simulink model "glucose"  (R2022a)
settings: Solver=VariableStepAuto  StartTime=0.0  StopTime=182  RelTol=1e-3
model workspace: external: MATLAB File parameters.m (data not in the file)
undefined symbols (not defined in the file): G0, Gb, Ib, insuline, k, Sg, Si, time
settings Model: Creator=bigba  LastModifiedBy=bigba

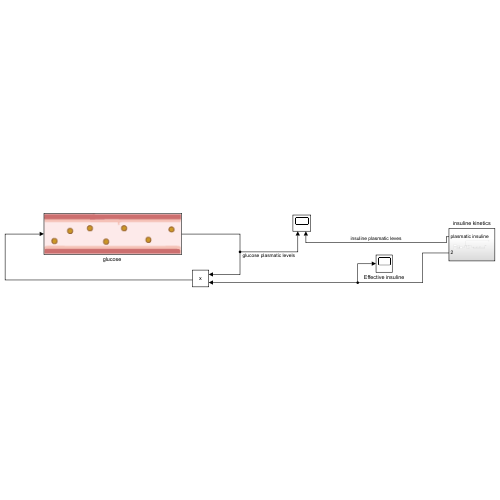
[thumbnail: Simulink's stored preview of the top-level diagram]
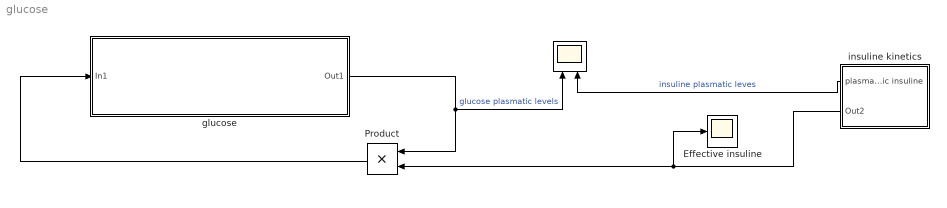
== system glucose ==
  " " : Scope  NumInputPorts=2
  Effective insuline : Scope
  Product : Product
  "glucose " : Subsystem
      mask Display: image('$imagefile'); % Use "Edit Image" on toolstrip to change.
  insuline kinetics : Subsystem
  wires:
  "glucose "/1(Out1) -> Product/1, " "/1  "glucose plasmatic levels"
  Product/1 -> "glucose "/1(In1)
  insuline kinetics/2(Out2) -> Product/2, Effective insuline/1
  insuline kinetics/1(plasmatic insuline) -> " "/2  "insuline plasmatic leves"

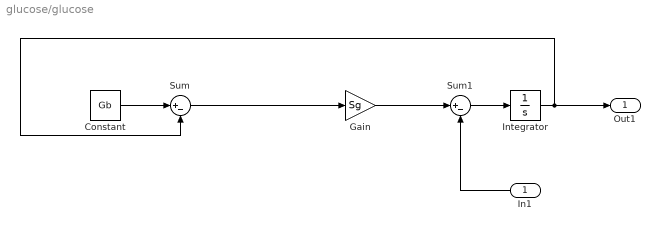
== system glucose/glucose  ==
  In1 : Inport
  Constant : Constant  Value=Gb
  Gain : Gain  Gain=Sg
  Integrator : Integrator  InitialCondition=G0
  Sum : Sum  Inputs=|+-
  Sum1 : Sum  Inputs=|+-
  Out1 : Outport
  wires:
  Gain/1 -> Sum1/1
  In1/1 -> Sum1/2
  Integrator/1 -> Out1/1, Sum/2
  Sum1/1 -> Integrator/1
  Constant/1 -> Sum/1
  Sum/1 -> Gain/1

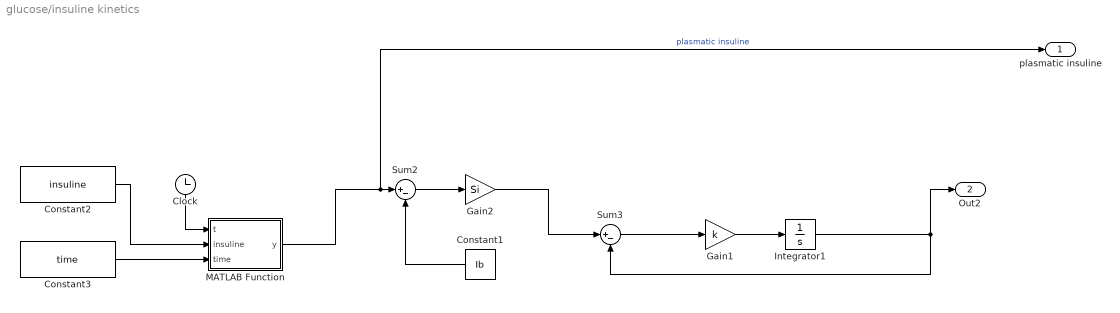
== system glucose/insuline kinetics ==
  Clock : Clock
  Constant1 : Constant  Value=Ib
  Constant2 : Constant  Value=insuline
  Constant3 : Constant  Value=time
  Gain1 : Gain  Gain=k
  Gain2 : Gain  Gain=Si
  Integrator1 : Integrator
  MATLAB Function : MATLAB Function  TreatAsAtomicUnit=on
  Sum2 : Sum  Inputs=|+-
  Sum3 : Sum  Inputs=|+-
  plasmatic insuline : Outport
  Out2 : Outport  Port=2
  wires:
  Gain1/1 -> Integrator1/1
  Sum2/1 -> Gain2/1
  Constant1/1 -> Sum2/2
  Integrator1/1 -> Out2/1, Sum3/2
  Sum3/1 -> Gain1/1
  Gain2/1 -> Sum3/1
  Clock/1 -> MATLAB Function/1(t)
  MATLAB Function/1(y) -> plasmatic insuline/1, Sum2/1  "plasmatic insuline"
  Constant3/1 -> MATLAB Function/3(time)
  Constant2/1 -> MATLAB Function/2(insuline)

== matlab function glucose/insuline kinetics/MATLAB Function ==
  data: t input; y output; insuline input; time input
function y = fcn(t,insuline,time)
y=interp1(time,insuline,t);
